simulink model "sampleModel292"  (R2021b)
settings: Solver=VariableStepAuto  StartTime=0.0  StopTime=10.0  RelTol=1e-3
libraries: simulink x3
settings Model: Creator=user  LastModifiedBy=user

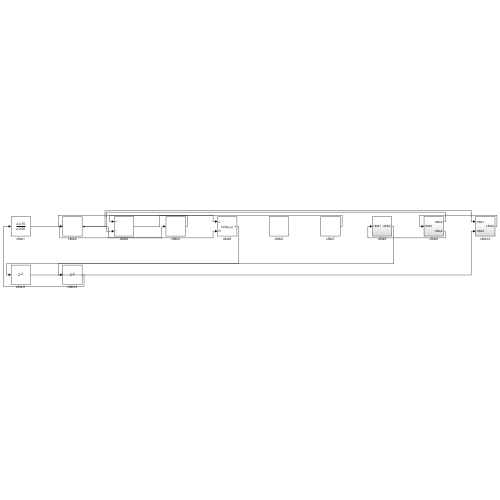
[thumbnail: Simulink's stored preview of the top-level diagram]
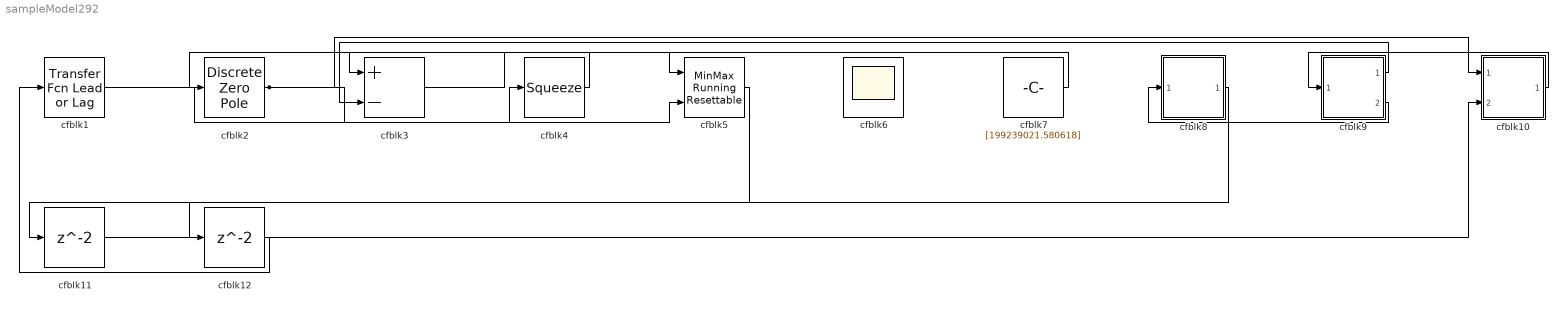
== system sampleModel292 ==
  cfblk1 : simulink/Discrete/Transfer Fcn Lead or Lag  PoleZ=0.95  ZeroZ=0.75  ICPrevOutput=0.0  ICPrevInput=0.0  DoSatur=off
      settings: SourceProductBaseCode=SL
  cfblk10 : Subsystem
  cfblk11 : Delay  SampleTime=1
  cfblk12 : Delay  SampleTime=1
  cfblk2 : DiscreteZeroPole  Poles=[0 0.5]  Gain=1
  cfblk3 : Sum  Inputs=+-
  cfblk4 : Squeeze
  cfblk5 : simulink/Math Operations/MinMax Running Resettable  Function=min  vinit=0.0
  cfblk6 : Scope
      settings: Floating=on
  cfblk7 : Constant  Value=[199239021.580618]  SampleTime=1
  cfblk8 : Subsystem
  cfblk9 : Subsystem
  wires:
  cfblk7/1 -> cfblk3/1
  cfblk1/1 -> cfblk4/1
  cfblk3/1 -> cfblk5/1
  cfblk9/1(cfblk2) -> cfblk3/2
  cfblk9/2(cfblk4) -> cfblk8/1(cfblk1)
  cfblk2/1 -> cfblk10/1(cfblk1), cfblk5/2
  cfblk10/1(cfblk2) -> cfblk9/1(cfblk1)
  cfblk4/1 -> cfblk2/1
  cfblk5/1 -> cfblk11/1
  cfblk11/1 -> cfblk10/2(cfblk3)
  cfblk8/1(cfblk2) -> cfblk12/1
  cfblk12/1 -> cfblk1/1

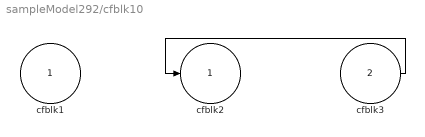
== system sampleModel292/cfblk10 ==
  cfblk1 : Inport
  cfblk3 : Inport  Port=2
  cfblk2 : Outport
  wires:
  cfblk3/1 -> cfblk2/1

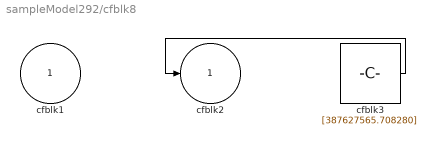
== system sampleModel292/cfblk8 ==
  cfblk1 : Inport
  cfblk3 : Constant  Value=[387627565.708280]  SampleTime=1
  cfblk2 : Outport
  wires:
  cfblk3/1 -> cfblk2/1

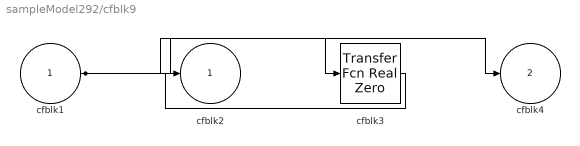
== system sampleModel292/cfblk9 ==
  cfblk1 : Inport
  cfblk3 : simulink/Discrete/Transfer Fcn Real Zero  ZeroZ=0.75  ICPrevInput=0.0  DoSatur=off
      settings: SourceProductBaseCode=SL
  cfblk2 : Outport
  cfblk4 : Outport  Port=2
  wires:
  cfblk1/1 -> cfblk4/1, cfblk3/1
  cfblk3/1 -> cfblk2/1
